simulink model "PMSM_FOC_SPEEDCUEEENTLOOP"  (R2022a)
settings: Solver=FixedStepAuto  StartTime=0.0  StopTime=10  FixedStep=Ts  RelTol=1e-3
values from neighbouring files (symbols this model uses):
  Ki_C = pmsm.Rs/(3*Ts)    [BR2804_1700Kv.m]
  Ki_S = (pi*pmsm.J)/(45*4*Ts*10^(2.5/2)*pmsm.p*pmsm.FluxPM*4*Ts*10^(2.5))    [BR2804_1700Kv.m]
  Kp_C = pmsm.Lq/(3*Ts)    [BR2804_1700Kv.m]
  Kp_S = (pi*pmsm.J)/(45*4*Ts*10^(2.5/2)*pmsm.p*pmsm.FluxPM)    [BR2804_1700Kv.m]
  Ts = T_pwm    (= 5e-05)    [BR2804_1700Kv.m]
undefined symbols (not defined in the file or in its folder): inverter, pmsm, sigbuilder_block
libraries: slpidlib x3, mcbplantlib x1, autolibpmsmexterior x1
settings Model: Creator=徐国强  LastModifiedBy=ZJH

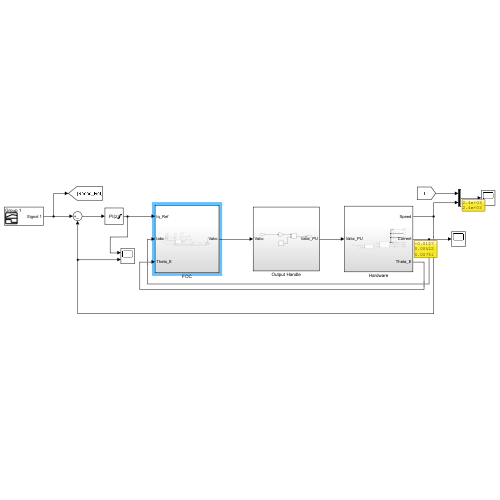
[thumbnail: Simulink's stored preview of the top-level diagram]
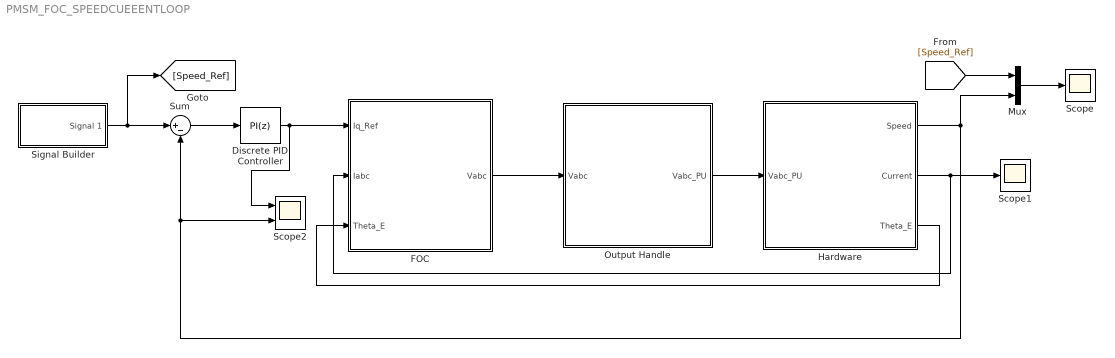
== system PMSM_FOC_SPEEDCUEEENTLOOP ==
  Discrete PID Controller : slpidlib/PID Controller  Controller=PI  Form=Parallel  TimeDomain=Discrete-time  UseExternalTs=off  SampleTime=-1  IntegratorMethod=Forward Euler  FilterMethod=Forward Euler  ControllerParametersSource=internal  P=Kp_S  I=Ki_S  UseKiTs=off  D=0  N=100  UseFilter=on  TunerSelectOption=Transfer Function Based (PID Tuner App)  InitialConditionSource=internal  InitialConditionForIntegrator=0  InitialConditionForFilter=0  DifferentiatorICPrevScaledInput=0  ExternalReset=none  TrackingMode=off  Kt=1  LimitOutput=on  SatLimitsSource=internal  UpperSaturationLimit=inverter.ISenseMax  LowerSaturationLimit=-inverter.ISenseMax  LinearizeAsGain=off  AntiWindupMode=none  Kb=1  POutMin=[]  POutMax=[]  IOutMin=[]  IOutMax=[]  DOutMin=[]  DOutMax=[]  NOutMin=[]  NOutMax=[]  SumOutMin=[]  SumOutMax=[]  SaturationOutMin=[]  SaturationOutMax=[]  PParamMin=[]  PParamMax=[]  IParamMin=[]  IParamMax=[]  DParamMin=[]  DParamMax=[]  NParamMin=[]  NParamMax=[]  KbParamMin=[]  KbParamMax=[]  KtParamMin=[]  KtParamMax=[]  KbOutMin=[]  KbOutMax=[]  KtOutMin=[]  KtOutMax=[]  IntegratorOutMin=[]  IntegratorOutMax=[]  FilterOutMin=[]  FilterOutMax=[]  SumI1OutMin=[]  SumI1OutMax=[]  SumI2OutMin=[]  SumI2OutMax=[]  SumI3OutMin=[]  SumI3OutMax=[]  SumI4OutMin=[]  SumI4OutMax=[]  SumDOutMin=[]  SumDOutMax=[]  DifferentiatorOutMin=[]  DifferentiatorOutMax=[]  FilterDiffOutCoefMin=[]  FilterDiffOutCoefMax=[]  ReciprocalOutMin=[]  ReciprocalOutMax=[]  SumDenOutMin=[]  SumDenOutMax=[]  SumNumOutMin=[]  SumNumOutMax=[]  DivideOutMin=[]  DivideOutMax=[]  UdiffTsProdOutMin=[]  UdiffTsProdOutMax=[]  NTsProdOutMin=[]  NTsProdOutMax=[]  UintegralTsProdOutMin=[]  UintegralTsProdOutMax=[]  UngainTsProdOutMin=[]  UngainTsProdOutMax=[]  IntegratorContinuousStateAttributes=''  IntegratorStateMustResolveToSignalObject=off  IntegratorRTWStateStorageClass=Auto  FilterContinuousStateAttributes=''  FilterStateMustResolveToSignalObject=off  FilterRTWStateStorageClass=Auto  ParallelPVariant=InternalParameters  IdealPVariant=Disabled  IVariant=InternalParameters  DVariant=Disabled  IntegratorVariant=Discrete  SatVariant=Enabled  AWVariant=Passthrough  PCopyVariant=Disabled  TRVariant=Disabled  FdbkBlocksVariant=Forward  IdealPFdbkVariant=Disabled  SatFdbkVariant=Disabled  DerivativeFilterVariant=Disabled  NVariant=Disabled  NCopyVariant=Disabled_SignalSpec  FilterICVariant=Disabled  IntegratorICVariant=InternalICs  ExternalResetVariant=Disabled  TRSumVariant=Passthrough  SumFdbkVariant=Disabled  SumVariant=Sum_PI  TsampFilterVariant=InternalTs  TsampNgainVariant=Passthrough  TsampIntegralVariant=Passthrough  ExternalSaturationOutDataTypeStr=Inherit: Same as second input  aMode=0
  FOC : Subsystem
  Hardware : Subsystem
  Mux : Mux  Inputs=2
  Output Handle : Subsystem
  Scope : Scope
  Scope1 : Scope
  Scope2 : Scope  NumInputPorts=2
  Signal Builder : Subsystem  Tag=STV Subsys  LoadFcn=sigbuilder_block('load');  StartFcn=sigbuilder_block('start');  StopFcn=sigbuilder_block('stop');  ClipboardFcn=sigbuilder_block('clipboard');  mask(Sigbuilder block){tuvar=[0:10]}
      mask help: Simulink:masks:SigbuilderBlock_MD
      mask init:
      | if ~strcmp(get_param(bdroot(gcbh),'SimulationStatus'),'stopped') tuvar = sigbuilder_block('maskInit'); end
      settings: CopyFcn=sigbuilder_block('copy');  DeleteFcn=sigbuilder_block('delete');  ModelCloseFcn=sigbuilder_block('modelClose');  PreSaveFcn=sigbuilder_block('preSave');  PauseFcn=sigbuilder_block('pause');  ContinueFcn=sigbuilder_block('continue');  NameChangeFcn=sigbuilder_block('namechange');  OpenFcn=sigbuilder_block('open',[437.6 199.2 550.4 400 ]);  CloseFcn=sigbuilder_block('close');
      mask Display: plot(0, 0, 100, 100,[2, 2, 32, 32, 2], [68, 8, 8, 68, 68],[32, 2], [38, 38], [32, 19, 2],[53, 60, 44], [32, 17, 17, 2],[16, 16, 31, 31]);txt = getActiveGroup(gcbh);text(2, 100, txt,'verticalAlignment', 'top');
  Sum : Sum  Inputs=|+-
  wires:
  Hardware/2(Current) -> FOC/2(Iabc), Scope1/1
  FOC/1(Vabc) -> Output Handle/1(Vabc)
  Output Handle/1(Vabc_PU) -> Hardware/1(Vabc_PU)
  Hardware/1(Speed) -> Mux/2, Scope2/2, Sum/2
  Sum/1 -> Discrete PID Controller/1
  Discrete PID Controller/1 -> Scope2/1, FOC/1(Iq_Ref)
  Hardware/3(Theta_E) -> FOC/3(Theta_E)
  Signal Builder/1(Signal 1) -> [Speed_Ref], Sum/1
  [Speed_Ref] -> Mux/1
  Mux/1 -> Scope/1

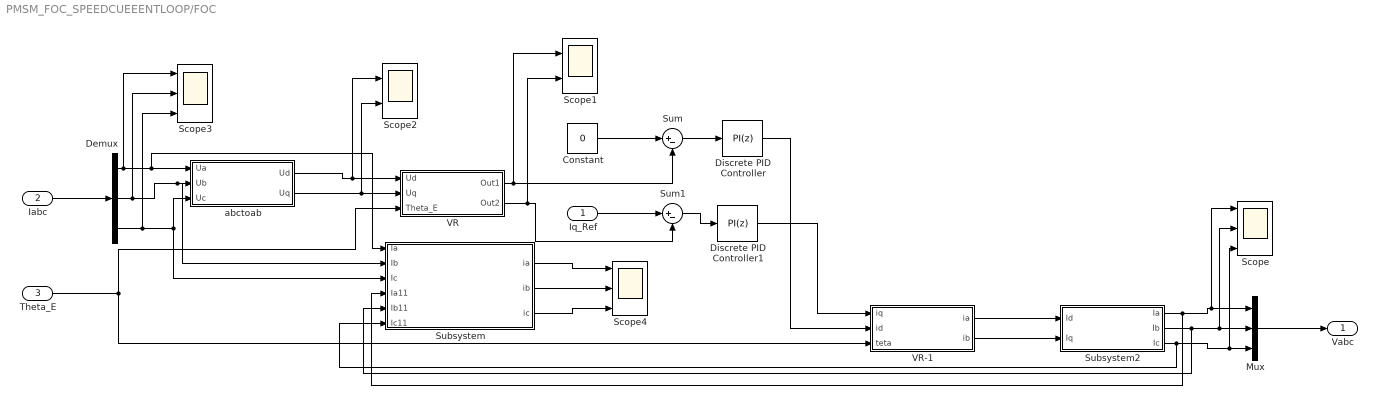
== system PMSM_FOC_SPEEDCUEEENTLOOP/FOC ==
  Iq_Ref : Inport
  Iabc : Inport  Port=2
  Theta_E : Inport  Port=3
  Constant : Constant  Value=0
  Demux : Demux  Outputs=3
  Discrete PID Controller : slpidlib/PID Controller  Controller=PI  Form=Parallel  TimeDomain=Discrete-time  UseExternalTs=off  SampleTime=-1  IntegratorMethod=Forward Euler  FilterMethod=Forward Euler  ControllerParametersSource=internal  P=Kp_C  I=Ki_C  UseKiTs=off  D=0  N=100  UseFilter=on  TunerSelectOption=Transfer Function Based (PID Tuner App)  InitialConditionSource=internal  InitialConditionForIntegrator=0  InitialConditionForFilter=0  DifferentiatorICPrevScaledInput=0  ExternalReset=none  TrackingMode=off  Kt=1  LimitOutput=on  SatLimitsSource=internal  UpperSaturationLimit=12/sqrt(3)  LowerSaturationLimit=-12/sqrt(3)  LinearizeAsGain=off  AntiWindupMode=none  Kb=1  POutMin=[]  POutMax=[]  IOutMin=[]  IOutMax=[]  DOutMin=[]  DOutMax=[]  NOutMin=[]  NOutMax=[]  SumOutMin=[]  SumOutMax=[]  SaturationOutMin=[]  SaturationOutMax=[]  PParamMin=[]  PParamMax=[]  IParamMin=[]  IParamMax=[]  DParamMin=[]  DParamMax=[]  NParamMin=[]  NParamMax=[]  KbParamMin=[]  KbParamMax=[]  KtParamMin=[]  KtParamMax=[]  KbOutMin=[]  KbOutMax=[]  KtOutMin=[]  KtOutMax=[]  IntegratorOutMin=[]  IntegratorOutMax=[]  FilterOutMin=[]  FilterOutMax=[]  SumI1OutMin=[]  SumI1OutMax=[]  SumI2OutMin=[]  SumI2OutMax=[]  SumI3OutMin=[]  SumI3OutMax=[]  SumI4OutMin=[]  SumI4OutMax=[]  SumDOutMin=[]  SumDOutMax=[]  DifferentiatorOutMin=[]  DifferentiatorOutMax=[]  FilterDiffOutCoefMin=[]  FilterDiffOutCoefMax=[]  ReciprocalOutMin=[]  ReciprocalOutMax=[]  SumDenOutMin=[]  SumDenOutMax=[]  SumNumOutMin=[]  SumNumOutMax=[]  DivideOutMin=[]  DivideOutMax=[]  UdiffTsProdOutMin=[]  UdiffTsProdOutMax=[]  NTsProdOutMin=[]  NTsProdOutMax=[]  UintegralTsProdOutMin=[]  UintegralTsProdOutMax=[]  UngainTsProdOutMin=[]  UngainTsProdOutMax=[]  IntegratorContinuousStateAttributes=''  IntegratorStateMustResolveToSignalObject=off  IntegratorRTWStateStorageClass=Auto  FilterContinuousStateAttributes=''  FilterStateMustResolveToSignalObject=off  FilterRTWStateStorageClass=Auto  ParallelPVariant=InternalParameters  IdealPVariant=Disabled  IVariant=InternalParameters  DVariant=Disabled  IntegratorVariant=Discrete  SatVariant=Enabled  AWVariant=Passthrough  PCopyVariant=Disabled  TRVariant=Disabled  FdbkBlocksVariant=Forward  IdealPFdbkVariant=Disabled  SatFdbkVariant=Disabled  DerivativeFilterVariant=Disabled  NVariant=Disabled  NCopyVariant=Disabled_SignalSpec  FilterICVariant=Disabled  IntegratorICVariant=InternalICs  ExternalResetVariant=Disabled  TRSumVariant=Passthrough  SumFdbkVariant=Disabled  SumVariant=Sum_PI  TsampFilterVariant=InternalTs  TsampNgainVariant=Passthrough  TsampIntegralVariant=Passthrough  ExternalSaturationOutDataTypeStr=Inherit: Same as second input  aMode=0
  Discrete PID Controller1 : slpidlib/PID Controller  Controller=PI  Form=Parallel  TimeDomain=Discrete-time  UseExternalTs=off  SampleTime=-1  IntegratorMethod=Forward Euler  FilterMethod=Forward Euler  ControllerParametersSource=internal  P=Kp_C  I=Ki_C  UseKiTs=off  D=0  N=100  UseFilter=on  TunerSelectOption=Transfer Function Based (PID Tuner App)  InitialConditionSource=internal  InitialConditionForIntegrator=0  InitialConditionForFilter=0  DifferentiatorICPrevScaledInput=0  ExternalReset=none  TrackingMode=off  Kt=1  LimitOutput=on  SatLimitsSource=internal  UpperSaturationLimit=12/sqrt(3)  LowerSaturationLimit=-12/sqrt(3)  LinearizeAsGain=off  AntiWindupMode=none  Kb=1  POutMin=[]  POutMax=[]  IOutMin=[]  IOutMax=[]  DOutMin=[]  DOutMax=[]  NOutMin=[]  NOutMax=[]  SumOutMin=[]  SumOutMax=[]  SaturationOutMin=[]  SaturationOutMax=[]  PParamMin=[]  PParamMax=[]  IParamMin=[]  IParamMax=[]  DParamMin=[]  DParamMax=[]  NParamMin=[]  NParamMax=[]  KbParamMin=[]  KbParamMax=[]  KtParamMin=[]  KtParamMax=[]  KbOutMin=[]  KbOutMax=[]  KtOutMin=[]  KtOutMax=[]  IntegratorOutMin=[]  IntegratorOutMax=[]  FilterOutMin=[]  FilterOutMax=[]  SumI1OutMin=[]  SumI1OutMax=[]  SumI2OutMin=[]  SumI2OutMax=[]  SumI3OutMin=[]  SumI3OutMax=[]  SumI4OutMin=[]  SumI4OutMax=[]  SumDOutMin=[]  SumDOutMax=[]  DifferentiatorOutMin=[]  DifferentiatorOutMax=[]  FilterDiffOutCoefMin=[]  FilterDiffOutCoefMax=[]  ReciprocalOutMin=[]  ReciprocalOutMax=[]  SumDenOutMin=[]  SumDenOutMax=[]  SumNumOutMin=[]  SumNumOutMax=[]  DivideOutMin=[]  DivideOutMax=[]  UdiffTsProdOutMin=[]  UdiffTsProdOutMax=[]  NTsProdOutMin=[]  NTsProdOutMax=[]  UintegralTsProdOutMin=[]  UintegralTsProdOutMax=[]  UngainTsProdOutMin=[]  UngainTsProdOutMax=[]  IntegratorContinuousStateAttributes=''  IntegratorStateMustResolveToSignalObject=off  IntegratorRTWStateStorageClass=Auto  FilterContinuousStateAttributes=''  FilterStateMustResolveToSignalObject=off  FilterRTWStateStorageClass=Auto  ParallelPVariant=InternalParameters  IdealPVariant=Disabled  IVariant=InternalParameters  DVariant=Disabled  IntegratorVariant=Discrete  SatVariant=Enabled  AWVariant=Passthrough  PCopyVariant=Disabled  TRVariant=Disabled  FdbkBlocksVariant=Forward  IdealPFdbkVariant=Disabled  SatFdbkVariant=Disabled  DerivativeFilterVariant=Disabled  NVariant=Disabled  NCopyVariant=Disabled_SignalSpec  FilterICVariant=Disabled  IntegratorICVariant=InternalICs  ExternalResetVariant=Disabled  TRSumVariant=Passthrough  SumFdbkVariant=Disabled  SumVariant=Sum_PI  TsampFilterVariant=InternalTs  TsampNgainVariant=Passthrough  TsampIntegralVariant=Passthrough  ExternalSaturationOutDataTypeStr=Inherit: Same as second input  aMode=0
  Mux : Mux  Inputs=3
  Scope : Scope  NumInputPorts=3
  Scope1 : Scope  NumInputPorts=2
  Scope2 : Scope  NumInputPorts=2
  Scope3 : Scope  NumInputPorts=3
  Scope4 : Scope  NumInputPorts=3
  Subsystem : Subsystem
  Subsystem2 : Subsystem
  Sum : Sum  Inputs=|+-
  Sum1 : Sum  Inputs=|+-
  VR : Subsystem
  VR-1 : Subsystem
  abctoab : Subsystem
  Vabc : Outport
  wires:
  Mux/1 -> Vabc/1
  Subsystem2/3(Ic) -> Subsystem/6(Ic11), Scope/3, Mux/3
  Subsystem2/2(Ib) -> Subsystem/5(Ib11), Scope/2, Mux/2
  Subsystem2/1(Ia) -> Subsystem/4(Ia11), Scope/1, Mux/1
  VR-1/2(ib) -> Subsystem2/2(Iq)
  VR-1/1(ia) -> Subsystem2/1(Id)
  Iabc/1 -> Demux/1
  Demux/1 -> Scope3/1, Subsystem/1(Ia), abctoab/1(Ua)
  Demux/3 -> Scope3/3, Subsystem/3(Ic), abctoab/3(Uc)
  abctoab/1(Ud) -> Scope2/1, VR/1(Ud)
  abctoab/2(Uq) -> Scope2/2, VR/2(Uq)
  Theta_E/1 -> VR-1/3(teta), VR/3(Theta_E)
  Constant/1 -> Sum/1
  VR/1(Out1) -> Scope1/1, Sum/2
  Iq_Ref/1 -> Sum1/1
  Sum/1 -> Discrete PID Controller/1
  Sum1/1 -> Discrete PID Controller1/1
  VR/2(Out2) -> Scope1/2, Sum1/2
  Discrete PID Controller1/1 -> VR-1/1(iq)
  Discrete PID Controller/1 -> VR-1/2(id)
  Demux/2 -> Scope3/2, Subsystem/2(Ib), abctoab/2(Ub)
  Subsystem/2(ib) -> Scope4/2
  Subsystem/1(ia) -> Scope4/1
  Subsystem/3(ic) -> Scope4/3

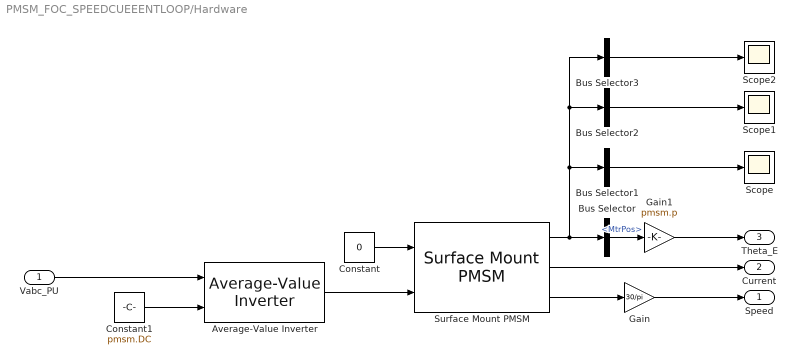
== system PMSM_FOC_SPEEDCUEEENTLOOP/Hardware ==
  Vabc_PU : Inport
  Average-Value Inverter : mcbplantlib/Average-Value Inverter
  Bus Selector : BusSelector  OutputSignals=MtrPos
  Bus Selector1 : BusSelector  OutputSignals=IdSync,IqSync  OutputAsBus=on
  Bus Selector2 : BusSelector  OutputSignals=VdSync,VqSync  OutputAsBus=on
  Bus Selector3 : BusSelector  OutputSignals=MtrTrq  OutputAsBus=on
  Constant : Constant  Value=0
  Constant1 : Constant  Value=pmsm.DC
  Gain : Gain  Gain=30/pi
  Gain1 : Gain  Gain=pmsm.p
  Scope : Scope
  Scope1 : Scope
  Scope2 : Scope
  Surface Mount PMSM : autolibpmsmexterior/Surface Mount PMSM  port_config=Torque  sim_type=Discrete  Ts=Ts  P=pmsm.p  Rs=pmsm.Rs  Ldq_=pmsm.Ld  KConstText=Permanent flux linkage constant (lambda_pm):  lambda_pm=pmsm.FluxPM  Ke=159.9771  Kt=1.323  mechanical=[pmsm.J, pmsm.B, 0]  idq0=[0 0]  theta_init=0  omega_init=0  KConst=pmsm.FluxPM  lambda_pm_calc=pmsm.FluxPM  RefBlkName='autolibpmsmexterior/Surface Mount PMSM'  aMode=5  Ldq="[0.0017      0.0017]"
      settings: SourceProductBaseCode=PW,DR,MT,VE
  Speed : Outport
  Current : Outport  Port=2
  Theta_E : Outport  Port=3
  wires:
  Vabc_PU/1 -> Average-Value Inverter/1
  Gain1/1 -> Theta_E/1
  Constant/1 -> Surface Mount PMSM/1
  Surface Mount PMSM/1 -> Bus Selector3/1, Bus Selector2/1, Bus Selector1/1, Bus Selector/1
  Surface Mount PMSM/3 -> Gain/1
  Average-Value Inverter/1 -> Surface Mount PMSM/2
  Surface Mount PMSM/2 -> Current/1
  Gain/1 -> Speed/1
  Constant1/1 -> Average-Value Inverter/2
  Bus Selector/1 -> Gain1/1  "<MtrPos>"
  Bus Selector1/1 -> Scope/1
  Bus Selector2/1 -> Scope1/1
  Bus Selector3/1 -> Scope2/1

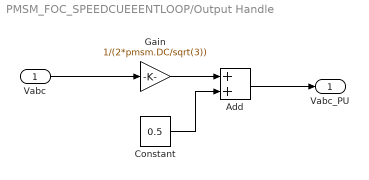
== system PMSM_FOC_SPEEDCUEEENTLOOP/Output Handle ==
  Vabc : Inport
  Add : Sum
  Constant : Constant  Value=0.5
  Gain : Gain  Gain=1/(2*pmsm.DC/sqrt(3))
  Vabc_PU : Outport
  wires:
  Constant/1 -> Add/2
  Add/1 -> Vabc_PU/1
  Gain/1 -> Add/1
  Vabc/1 -> Gain/1

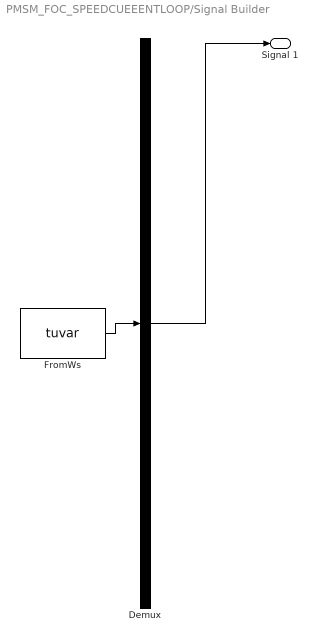
== system PMSM_FOC_SPEEDCUEEENTLOOP/Signal Builder ==
  Demux : Demux  Tag=STV Demux  Outputs=1
      settings: DisplayOption=none
  FromWs : FromWorkspace  Tag=STV FromWs  VariableName=tuvar
      SigBuilderData=|
      | common.afterFinalStr = 'Extrapolate'
      | common.sampleTime = 0
      | dataSet.timeRange = [0 10]
      | dataSet.name = 'Group 1'
      | sbobj.Groups.Name = 'Group 1'
      | sbobj.Groups.Signals.Name = 'Signal 1'
      | sbobj.Groups.Signals.XData = [0 2 2 4 4 6 6 7.98 7.98 10]
      | sbobj.Groups.Signals.YData = [1200 1200 2100 2100 3800 3800 6100 6100 2400 2400]
  Signal 1 : Outport  Tag=STV Outport
  wires:
  Demux/1 -> Signal 1/1
  FromWs/1 -> Demux/1

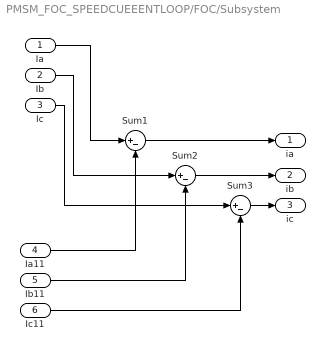
== system PMSM_FOC_SPEEDCUEEENTLOOP/FOC/Subsystem ==
  Ia : Inport
  Ib : Inport  Port=2
  Ic : Inport  Port=3
  Ia11 : Inport  Port=4
  Ib11 : Inport  Port=5
  Ic11 : Inport  Port=6
  Sum1 : Sum  Inputs=|+-
  Sum2 : Sum  Inputs=|+-
  Sum3 : Sum  Inputs=|+-
  ia : Outport
  ib : Outport  Port=2
  ic : Outport  Port=3
  wires:
  Sum3/1 -> ic/1
  Sum2/1 -> ib/1
  Sum1/1 -> ia/1
  Ia/1 -> Sum1/1
  Ia11/1 -> Sum1/2
  Ib/1 -> Sum2/1
  Ib11/1 -> Sum2/2
  Ic/1 -> Sum3/1
  Ic11/1 -> Sum3/2

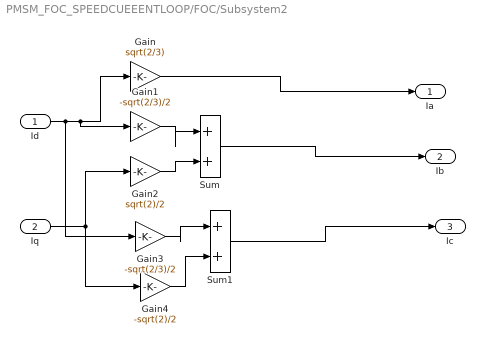
== system PMSM_FOC_SPEEDCUEEENTLOOP/FOC/Subsystem2 ==
  Id : Inport
  Iq : Inport  Port=2
  Gain : Gain  Gain=sqrt(2/3)  SaturateOnIntegerOverflow=on  OutDataTypeStr=Inherit: Same as input  ParamDataTypeStr=Inherit: Same as input
  Gain1 : Gain  Gain=-sqrt(2/3)/2  SaturateOnIntegerOverflow=on  OutDataTypeStr=Inherit: Same as input  ParamDataTypeStr=Inherit: Same as input
  Gain2 : Gain  Gain=sqrt(2)/2  SaturateOnIntegerOverflow=on  OutDataTypeStr=Inherit: Same as input  ParamDataTypeStr=Inherit: Same as input
  Gain3 : Gain  Gain=-sqrt(2/3)/2  SaturateOnIntegerOverflow=on  OutDataTypeStr=Inherit: Same as input  ParamDataTypeStr=Inherit: Same as input
  Gain4 : Gain  Gain=-sqrt(2)/2  SaturateOnIntegerOverflow=on  OutDataTypeStr=Inherit: Same as input  ParamDataTypeStr=Inherit: Same as input
  Sum : Sum  Inputs=|++  SaturateOnIntegerOverflow=on
  Sum1 : Sum  Inputs=|++  SaturateOnIntegerOverflow=on
  Ia : Outport
  Ib : Outport  Port=2
  Ic : Outport  Port=3
  wires:
  Id/1 -> Gain/1, Gain1/1, Gain3/1
  Gain/1 -> Ia/1
  Iq/1 -> Gain2/1, Gain4/1
  Gain1/1 -> Sum/1
  Gain2/1 -> Sum/2
  Sum/1 -> Ib/1
  Gain3/1 -> Sum1/1
  Gain4/1 -> Sum1/2
  Sum1/1 -> Ic/1

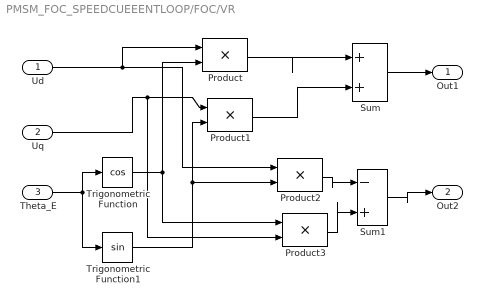
== system PMSM_FOC_SPEEDCUEEENTLOOP/FOC/VR ==
  Ud : Inport
  Uq : Inport  Port=2
  Theta_E : Inport  Port=3
  Product{,1..3} (4 alike) : Product  SaturateOnIntegerOverflow=on  OutDataTypeStr=Inherit: Same as first input
  Sum : Sum  Inputs=|++  SaturateOnIntegerOverflow=on
  Sum1 : Sum  Inputs=|-+  SaturateOnIntegerOverflow=on
  Trigonometric Function : Trigonometry  Operator=cos
  Trigonometric Function1 : Trigonometry
  Out1 : Outport
  Out2 : Outport  Port=2
  wires:
  Product3/1 -> Sum1/2
  Product2/1 -> Sum1/1
  Product1/1 -> Sum/2
  Uq/1 -> Product3/2, Product1/1
  Trigonometric Function1/1 -> Product2/2, Product1/2
  Product/1 -> Sum/1
  Trigonometric Function/1 -> Product3/1, Product/2
  Ud/1 -> Product2/1, Product/1
  Sum1/1 -> Out2/1
  Theta_E/1 -> Trigonometric Function1/1, Trigonometric Function/1
  Sum/1 -> Out1/1

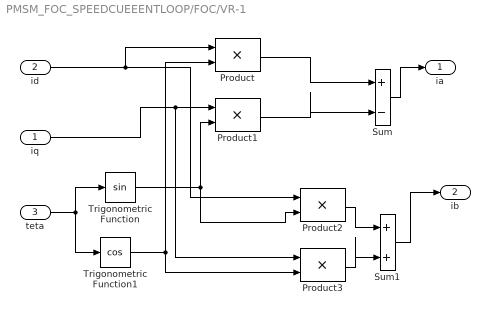
== system PMSM_FOC_SPEEDCUEEENTLOOP/FOC/VR-1 ==
  iq : Inport
  id : Inport  Port=2
  teta : Inport  Port=3
  Product{,1..3} (4 alike) : Product  SaturateOnIntegerOverflow=on  OutDataTypeStr=Inherit: Same as first input
  Sum : Sum  Inputs=|+-  SaturateOnIntegerOverflow=on
  Sum1 : Sum  Inputs=|++  SaturateOnIntegerOverflow=on
  Trigonometric Function : Trigonometry
  Trigonometric Function1 : Trigonometry  Operator=cos
  ia : Outport
  ib : Outport  Port=2
  wires:
  Sum1/1 -> ib/1
  Product3/1 -> Sum1/2
  Product2/1 -> Sum1/1
  Sum/1 -> ia/1
  Product1/1 -> Sum/2
  iq/1 -> Product3/1, Product1/1
  Trigonometric Function/1 -> Product2/2, Product1/2
  Product/1 -> Sum/1
  Trigonometric Function1/1 -> Product3/2, Product/2
  id/1 -> Product2/1, Product/1
  teta/1 -> Trigonometric Function1/1, Trigonometric Function/1

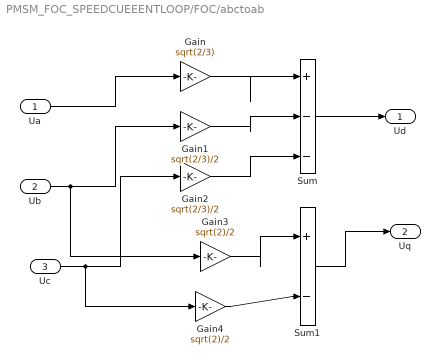
== system PMSM_FOC_SPEEDCUEEENTLOOP/FOC/abctoab ==
  Ua : Inport
  Ub : Inport  Port=2
  Uc : Inport  Port=3
  Gain : Gain  Gain=sqrt(2/3)  SaturateOnIntegerOverflow=on  OutDataTypeStr=Inherit: Same as input  ParamDataTypeStr=Inherit: Same as input
  Gain1 : Gain  Gain=sqrt(2/3)/2  SaturateOnIntegerOverflow=on  OutDataTypeStr=Inherit: Same as input  ParamDataTypeStr=Inherit: Same as input
  Gain2 : Gain  Gain=sqrt(2/3)/2  SaturateOnIntegerOverflow=on  OutDataTypeStr=Inherit: Same as input  ParamDataTypeStr=Inherit: Same as input
  Gain3 : Gain  Gain=sqrt(2)/2  SaturateOnIntegerOverflow=on  OutDataTypeStr=Inherit: Same as input  ParamDataTypeStr=Inherit: Same as input
  Gain4 : Gain  Gain=sqrt(2)/2  SaturateOnIntegerOverflow=on  OutDataTypeStr=Inherit: Same as input  ParamDataTypeStr=Inherit: Same as input
  Sum : Sum  Inputs=|+--  SaturateOnIntegerOverflow=on
  Sum1 : Sum  Inputs=|+-  SaturateOnIntegerOverflow=on
  Ud : Outport
  Uq : Outport  Port=2
  wires:
  Sum1/1 -> Uq/1
  Gain4/1 -> Sum1/2
  Gain3/1 -> Sum1/1
  Sum/1 -> Ud/1
  Gain2/1 -> Sum/3
  Gain1/1 -> Sum/2
  Gain/1 -> Sum/1
  Uc/1 -> Gain4/1, Gain2/1
  Ub/1 -> Gain3/1, Gain1/1
  Ua/1 -> Gain/1
